simulink model "CC_m3"  (R2020b)
settings: Solver=ode3  StartTime=0.0  StopTime=simTime  FixedStep=0.001  RelTol=1e-3
undefined symbols (not defined in the file): DiscIntNeverNeededParam, Kdec, KInc, Kp, Kp1
settings Model: LastModifiedBy=Xiao Ling
settings DataIOCC: SaveFormat=Array  SignalLogging=off  DSMLogging=off  ReturnWorkspaceOutputs=off
settings OptimizationCC: LifeSpan=inf
settings DebuggingCC: UnderspecifiedInitializationDetection=Classic  MergeDetectMultiDrivingBlocksExec=none  SolverPrmCheckMsg=warning  StateNameClashWarn=warning  SFUnexpectedBacktrackingDiag=warning  SFNoUnconditionalDefaultTransitionDiag=warning  SFExecutionAtInitializationDiag=none  ArithmeticOperatorsInVariantConditions=warning
settings HardwareCC: ProdBitPerPointer=32  ProdBitPerSizeT=32  ProdBitPerPtrDiffT=32  ProdLargestAtomicFloat=None  ProdIntDivRoundTo=Undefined  ProdEndianess=Unspecified  ProdWordSize=32  ProdHWDeviceType=32-bit Generic
settings ModelReferenceCC: PropagateSignalLabelsOutOfModel=off
settings SFSimCC: SimUseLocalCustomCode=off  CustomCodeUndefinedFunction=UseInterfaceOnly
settings RTWCC: RTWUseLocalCustomCode=off
settings CodeAppCC: StateflowObjectComments=on
settings GRTTargetCC: TargetLangStandard=C89/C90 (ANSI)
settings ConfigComp: CovMetricSettings=dw  CovSaveCumulativeToWorkspaceVar=on  CovSaveSingleToWorkspaceVar=on  CovExternalEMLEnable=off

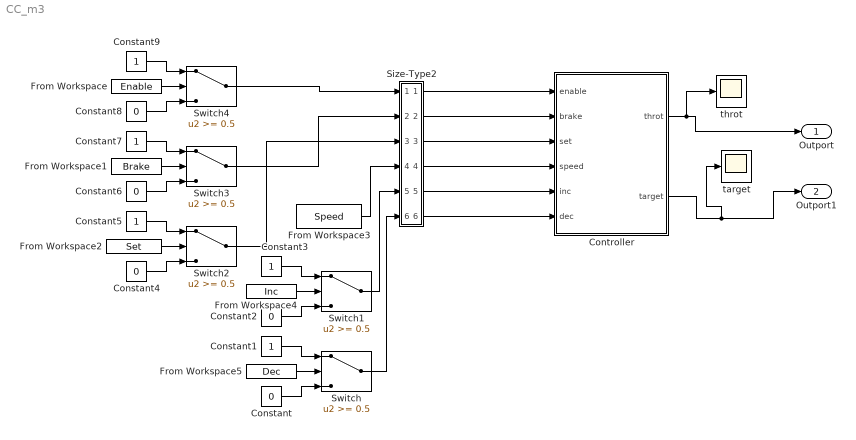
== system CC_m3 ==
  Constant{,2,4,6,8} (5 alike) : Constant  Value=0
  Constant{1,3,5,7,9} (5 alike) : Constant
  Controller : Subsystem
  From Workspace : FromWorkspace  VariableName=Enable
  From Workspace1 : FromWorkspace  VariableName=Brake
  From Workspace2 : FromWorkspace  VariableName=Set
  From Workspace3 : FromWorkspace  VariableName=Speed
  From Workspace4 : FromWorkspace  VariableName=Inc
  From Workspace5 : FromWorkspace  VariableName=Dec
  Size-Type2 : Subsystem
  Switch{,1..4} (5 alike) : Switch  Threshold=0.5
  target : Scope
  throt : Scope
  Outport : Outport
  Outport1 : Outport  Port=2
  wires:
  From Workspace3/1 -> Size-Type2/4(In4)
  From Workspace5/1 -> Switch/2
  Size-Type2/1(Out1) -> Controller/1(enable)
  Size-Type2/3(Out3) -> Controller/3(set)
  Size-Type2/5(Out5) -> Controller/5(inc)
  Size-Type2/6(Out6) -> Controller/6(dec)
  Size-Type2/4(Out4) -> Controller/4(speed)
  Size-Type2/2(Out2) -> Controller/2(brake)
  Controller/2(target) -> target/1, Outport1/1
  Controller/1(throt) -> throt/1, Outport/1
  Constant1/1 -> Switch/1
  Constant/1 -> Switch/3
  Switch/1 -> Size-Type2/6(In6)
  Constant3/1 -> Switch1/1
  Constant2/1 -> Switch1/3
  From Workspace4/1 -> Switch1/2
  Switch1/1 -> Size-Type2/5(In5)
  From Workspace2/1 -> Switch2/2
  Constant4/1 -> Switch2/3
  Constant5/1 -> Switch2/1
  Switch2/1 -> Size-Type2/3(In3)
  From Workspace1/1 -> Switch3/2
  Constant6/1 -> Switch3/3
  Constant7/1 -> Switch3/1
  Switch3/1 -> Size-Type2/2(In2)
  From Workspace/1 -> Switch4/2
  Constant8/1 -> Switch4/3
  Constant9/1 -> Switch4/1
  Switch4/1 -> Size-Type2/1(In1)

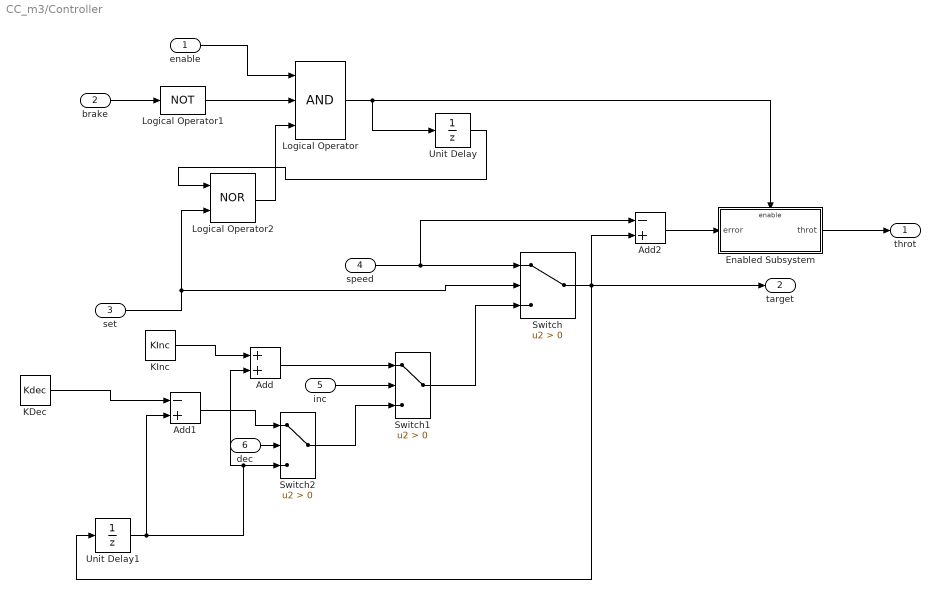
== system CC_m3/Controller ==
  enable : Inport
  brake : Inport  Port=2
  set : Inport  Port=3
  speed : Inport  Port=4
  inc : Inport  Port=5
  dec : Inport  Port=6
  Add : Sum
  Add1 : Sum  Inputs=-+
  Add2 : Sum  Inputs=-+
  Enabled Subsystem : Subsystem  TreatAsAtomicUnit=on
  KDec : Constant  Value=Kdec
  KInc : Constant  Value=KInc
  Logical Operator : Logic  Inputs=3  AllPortsSameDT=off  OutDataTypeStr=boolean
  Logical Operator1 : Logic  Operator=NOT  Inputs=3  AllPortsSameDT=off  OutDataTypeStr=boolean
  Logical Operator2 : Logic  Operator=NOR  AllPortsSameDT=off  OutDataTypeStr=boolean
  Switch : Switch  Criteria=u2 > Threshold
  Switch1 : Switch  Criteria=u2 > Threshold
  Switch2 : Switch  Criteria=u2 > Threshold
  Unit Delay : UnitDelay  InitialCondition=1  SampleTime=-1  HasFrameUpgradeWarning=on
  Unit Delay1 : UnitDelay  SampleTime=-1  HasFrameUpgradeWarning=on
  throt : Outport  VectorParamsAs1DForOutWhenUnconnected=off
  target : Outport  Port=2  VectorParamsAs1DForOutWhenUnconnected=off
  wires:
  enable/1 -> Logical Operator/1
  Logical Operator1/1 -> Logical Operator/2
  brake/1 -> Logical Operator1/1
  set/1 -> Logical Operator2/2, Switch/2
  Logical Operator/1 -> Enabled Subsystem/Enable, Unit Delay/1
  Unit Delay/1 -> Logical Operator2/1
  Logical Operator2/1 -> Logical Operator/3
  speed/1 -> Add2/1, Switch/1
  Switch1/1 -> Switch/3
  Switch2/1 -> Switch1/3
  Add/1 -> Switch1/1
  inc/1 -> Switch1/2
  dec/1 -> Switch2/2
  Switch/1 -> target/1, Add2/2, Unit Delay1/1
  Unit Delay1/1 -> Add1/2, Add/2, Switch2/3
  KInc/1 -> Add/1
  Add1/1 -> Switch2/1
  KDec/1 -> Add1/1
  Add2/1 -> Enabled Subsystem/1(error)
  Enabled Subsystem/1(throt) -> throt/1

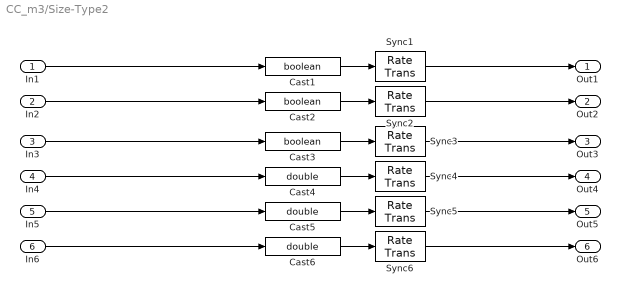
== system CC_m3/Size-Type2 ==
  In1 : Inport
  In2 : Inport  Port=2
  In3 : Inport  Port=3
  In4 : Inport  Port=4
  In5 : Inport  Port=5
  In6 : Inport  Port=6
  Cast1 : DataTypeConversion  OutDataTypeStr=boolean  SaturateOnIntegerOverflow=on  RndMeth=Zero
  Cast2 : DataTypeConversion  OutDataTypeStr=boolean  SaturateOnIntegerOverflow=on  RndMeth=Zero
  Cast3 : DataTypeConversion  OutDataTypeStr=boolean  SaturateOnIntegerOverflow=on  RndMeth=Zero
  Cast4 : DataTypeConversion  OutDataTypeStr=double  SaturateOnIntegerOverflow=on  RndMeth=Zero
  Cast5 : DataTypeConversion  OutDataTypeStr=double  SaturateOnIntegerOverflow=on  RndMeth=Zero
  Cast6 : DataTypeConversion  OutDataTypeStr=double  SaturateOnIntegerOverflow=on  RndMeth=Zero
  Sync{1..6} (6 alike) : RateTransition  OutPortSampleTime=[1,0]
  Out1 : Outport  VectorParamsAs1DForOutWhenUnconnected=off
  Out2 : Outport  Port=2  VectorParamsAs1DForOutWhenUnconnected=off
  Out3 : Outport  Port=3  VectorParamsAs1DForOutWhenUnconnected=off
  Out4 : Outport  Port=4  VectorParamsAs1DForOutWhenUnconnected=off
  Out5 : Outport  Port=5  VectorParamsAs1DForOutWhenUnconnected=off
  Out6 : Outport  Port=6  VectorParamsAs1DForOutWhenUnconnected=off
  wires:
  Sync6/1 -> Out6/1
  Cast6/1 -> Sync6/1
  In6/1 -> Cast6/1
  Sync5/1 -> Out5/1
  Cast5/1 -> Sync5/1
  In5/1 -> Cast5/1
  Sync4/1 -> Out4/1
  Cast4/1 -> Sync4/1
  In4/1 -> Cast4/1
  Sync3/1 -> Out3/1
  Cast3/1 -> Sync3/1
  In3/1 -> Cast3/1
  Sync2/1 -> Out2/1
  Cast2/1 -> Sync2/1
  In2/1 -> Cast2/1
  Sync1/1 -> Out1/1
  Cast1/1 -> Sync1/1
  In1/1 -> Cast1/1

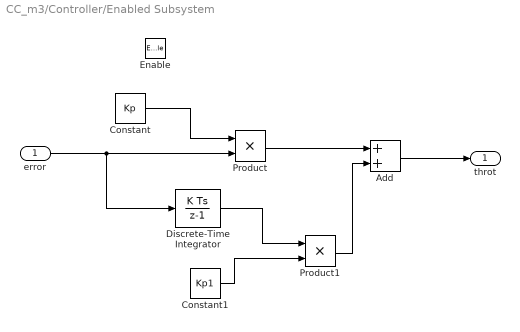
== system CC_m3/Controller/Enabled Subsystem ==
  error : Inport
  Enable : EnablePort
  Add : Sum
  Constant : Constant  Value=Kp
  Constant1 : Constant  Value=Kp1
  Discrete-Time Integrator : DiscreteIntegrator  gainval=Ki  ICPrevOutput=DiscIntNeverNeededParam  ICPrevScaledInput=DiscIntNeverNeededParam
  Product : Product
  Product1 : Product
  throt : Outport  VectorParamsAs1DForOutWhenUnconnected=off
  wires:
  Constant/1 -> Product/1
  Product/1 -> Add/1
  Add/1 -> throt/1
  Constant1/1 -> Product1/2
  Product1/1 -> Add/2
  Discrete-Time Integrator/1 -> Product1/1
  error/1 -> Discrete-Time Integrator/1, Product/2
